simulink model "cal_length_norm_2d"  (R2017b)
settings: Solver=FixedStepAuto  StartTime=0.0  StopTime=5  FixedStep=dt  RelTol=1e-3
settings Model: Creator=af  LastModifiedBy=af
settings DataIOCC: SaveOutput=off  SaveTime=off

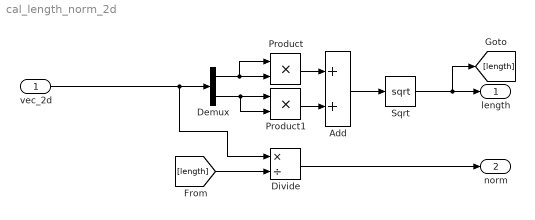
== system cal_length_norm_2d ==
  vec_2d : Inport  OutDataTypeStr=double  PortDimensions=2  SampleTime=0
  Add : Sum
  Demux : Demux  Outputs=2
  Divide : Product  Inputs=*/
  Product : Product
  Product1 : Product
  Sqrt : Sqrt  SaturateOnIntegerOverflow=on
  length : Outport  OutDataTypeStr=double  PortDimensions=1  SampleTime=0
  norm : Outport  Port=2  OutDataTypeStr=double  PortDimensions=2  SampleTime=0
  wires:
  [length] -> Divide/2
  Demux/2 -> Product1/1, Product1/2
  Product/1 -> Add/1
  Divide/1 -> norm/1
  vec_2d/1 -> Demux/1, Divide/1
  Add/1 -> Sqrt/1
  Demux/1 -> Product/2, Product/1
  Product1/1 -> Add/2
  Sqrt/1 -> [length], length/1
